simulink model "px4demo_uORBReadWrite"  (R2019b)
settings: Solver=FixedStepAuto  StartTime=0.0  StopTime=inf  RelTol=1e-3  EnableMultiTasking=on
undefined symbols (not defined in the file or in its folder): alt, lat, lon, vel_m_s
libraries: px4uORBlib x3
settings Model: SimulationMode=external  ExtModeTrigDuration=10  Creator=The MathWorks, Inc.  LastModifiedBy=The MathWorks, Inc.
settings SolverCC: PositivePriorityOrder=on
settings OptimizationCC: EnhancedBackFolding=on  PassReuseOutputArgsAs=Individual arguments  ZeroExternalMemoryAtStartup=off  ZeroInternalMemoryAtStartup=off  MaxStackSize=64  OptimizeBlockOrder=speed  DifferentSizesBufferReuse=on  OptimizationCustomize=off  EfficientTunableParamExpr=on
settings DebuggingCC: ParameterTunabilityLossMsg=error
settings HardwareCC: ProdBitPerPointer=32  ProdBitPerSizeT=32  ProdBitPerPtrDiffT=32  ProdLargestAtomicInteger=Long  ProdLargestAtomicFloat=Double  ProdWordSize=32  ProdLongLongMode=on  ProdHWDeviceType=ARM Compatible->ARM Cortex
settings SFSimCC: MATLABDynamicMemAlloc=off
settings RTWCC: SystemTargetFile=ert.tlc  HardwareBoard=PX4 Pixhawk 1  TLCOptions="-aInlineSetEventsForThisBaseRateFcn=TLC_FALSE -aSuppressMultiTaskScheduler=TLC_FALSE  -aRateBasedStepFcn=0"  TemplateMakefile=ert_default_tmf  GenerateReport=on  Toolchain=GNU Tools for PX4 Autopilots  IncludeHyperlinkInReport=on  LaunchReport=on  TargetLang=C++  GenerateTraceInfo=on  GenerateTraceReport=on  GenerateTraceReportSl=on  GenerateTraceReportSf=on  GenerateTraceReportEml=on
settings CodeAppCC: ForceParamTrailComments=on  IgnoreCustomStorageClasses=off  OperatorAnnotations=on  SimulinkDataObjDesc=on  SFDataObjDesc=on  InsertBlockDesc=on

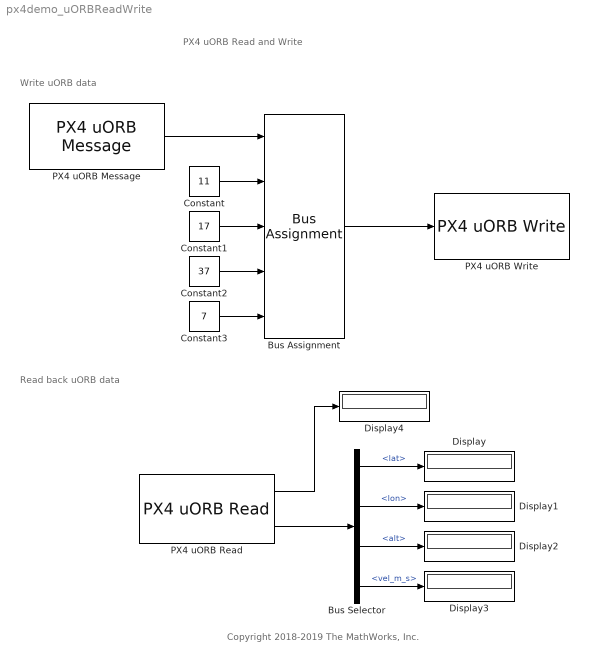
== system px4demo_uORBReadWrite ==
  note: Copyright 2018-2019 The MathWorks, Inc.
  note: PX4 uORB Read and Write
  note: Write uORB data
  note: Read back uORB data
  Bus Assignment : BusAssignment  AssignedSignals=lat,lon,alt,vel_m_s
  Bus Selector : BusSelector  OutputSignals=lat,lon,alt,vel_m_s
  Constant : Constant  Value=11  OutDataTypeStr=Inherit: Inherit via back propagation  SampleTime=0.1
  Constant1 : Constant  Value=17  OutDataTypeStr=Inherit: Inherit via back propagation  SampleTime=0.1
  Constant2 : Constant  Value=37  OutDataTypeStr=Inherit: Inherit via back propagation  SampleTime=0.1
  Constant3 : Constant  Value=7  OutDataTypeStr=Inherit: Inherit via back propagation  SampleTime=0.1
  Display{,1..4} (5 alike) : Display
  PX4 uORB Message : px4uORBlib/PX4 uORB Message  uORBTopic=vehicle_gps_position  SampleTime=inf
      settings: SourceProductName=Embedded Coder Support Package for PX4 Autopilots  SourceProductBaseCode=PX4AUTOPILOTS
  PX4 uORB Read : px4uORBlib/PX4 uORB Read  uORBTopic=vehicle_gps_position  sampleTime=0.1  BlockingMode=off  BlockTimeout=1e-3
      settings: SourceProductName=Embedded Coder Support Package for PX4 Autopilots  SourceProductBaseCode=PX4AUTOPILOTS
  PX4 uORB Write : px4uORBlib/PX4 uORB Write  uORBTopic=vehicle_gps_position  MessageQueueLen=1
      settings: SourceProductName=Embedded Coder Support Package for PX4 Autopilots  SourceProductBaseCode=PX4AUTOPILOTS
  wires:
  PX4 uORB Message/1 -> Bus Assignment/1
  Bus Assignment/1 -> PX4 uORB Write/1
  Constant/1 -> Bus Assignment/2
  Constant1/1 -> Bus Assignment/3
  Constant2/1 -> Bus Assignment/4
  Constant3/1 -> Bus Assignment/5
  PX4 uORB Read/2 -> Bus Selector/1
  Bus Selector/1 -> Display/1  "<lat>"
  Bus Selector/2 -> Display1/1  "<lon>"
  Bus Selector/3 -> Display2/1  "<alt>"
  Bus Selector/4 -> Display3/1  "<vel_m_s>"
  PX4 uORB Read/1 -> Display4/1
